simulink model "a6_real_test"  (R2023b)
settings: Solver=FixedStepAuto  StartTime=0.0  StopTime=inf  RelTol=1e-3  EnableMultiTasking=on
undefined symbols (not defined in the file): dev, Main, pwm_output0
libraries: simulink x4, px4Sensorslib x3, px4lib x1, px4uORBlib x1
settings Model: ExtModeTrigDuration=10  Creator=UAV2  LastModifiedBy=UAV2
settings SolverCC: AlgebraicLoopSolver=TrustRegion  PositivePriorityOrder=on  MaxZcPerStep=1
settings OptimizationCC: EnhancedBackFolding=on  PassReuseOutputArgsAs=Individual arguments  ZeroExternalMemoryAtStartup=off  ZeroInternalMemoryAtStartup=off  MaxStackSize=64  OptimizeBlockOrder=speed  DifferentSizesBufferReuse=on  OptimizationCustomize=off  EfficientTunableParamExpr=on
settings DebuggingCC: ParameterTunabilityLossMsg=error  UnconnectedInputMsg=warning  UnconnectedOutputMsg=warning  UnconnectedLineMsg=warning  SymbolicDimsDataTypeCodeGenerationDiagnostic=none
settings HardwareCC: ProdBitPerPointer=32  ProdBitPerSizeT=32  ProdBitPerPtrDiffT=32  ProdLargestAtomicInteger=Long  ProdLargestAtomicFloat=Double  ProdWordSize=32  ProdLongLongMode=on  ProdHWDeviceType=ARM Compatible->ARM Cortex
settings ModelReferenceCC: EnableRefExpFcnMdlSchedulingChecks=on
settings SFSimCC: MATLABDynamicMemAlloc=off  SimTargetLang=C++
settings RTWCC: Description=Embedded Coder  SystemTargetFile=ert.tlc  HardwareBoard=PX4 Pixhawk 4  TLCOptions="-aInlineSetEventsForThisBaseRateFcn=TLC_FALSE -aSuppressMultiTaskScheduler=TLC_FALSE  -aRateBasedStepFcn=0"  TemplateMakefile=ert_default_tmf  Toolchain=GNU Tools for PX4 Autopilots  IncludeHyperlinkInReport=on  TargetLang=C++  DLArmComputeVersion=19.05
settings CodeAppCC: ForceParamTrailComments=on  IgnoreCustomStorageClasses=off  OperatorAnnotations=on  SimulinkDataObjDesc=on  SFDataObjDesc=on  InsertBlockDesc=on
settings ERTTargetCC: ExtModeTransport=3  ExtModeStaticAlloc=on  ExtModeStaticAllocSize=1024  ExtModeMexFile=ext_xcp  ExtModeIntrfLevel=Level2 - Open

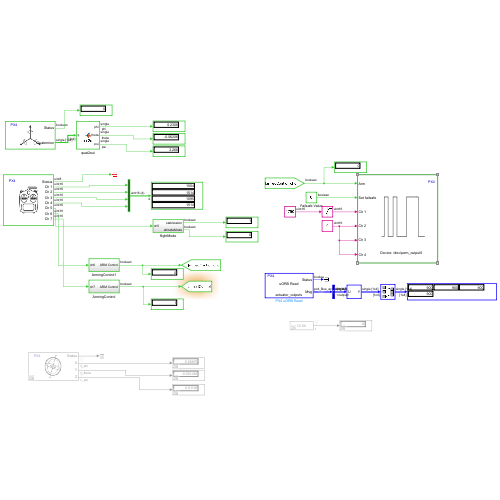
[thumbnail: Simulink's stored preview of the top-level diagram]
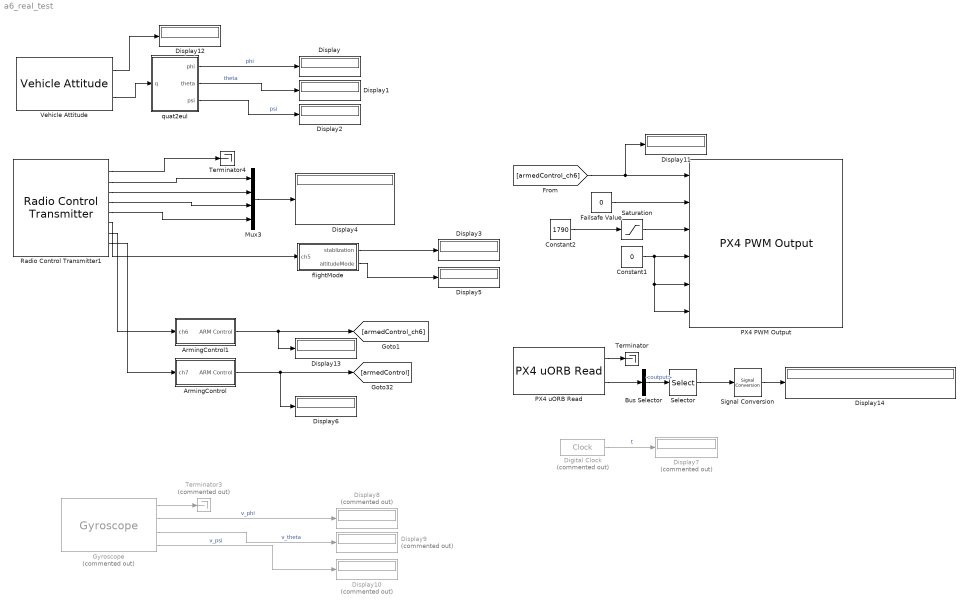
== system a6_real_test ==
  ArmingControl : Subsystem
  ArmingControl1 : Subsystem
  Bus Selector : BusSelector  OutputSignals=output
  Constant1 : Constant  Value=0  OutDataTypeStr=uint16
  Constant2 : Constant  Value=1790  OutDataTypeStr=uint16
  Digital Clock : DigitalClock  Commented=on
  Display{,1..6,11..14} (11 alike) : Display
      Display4 settings: Format=decimal (Stored Integer)
  Display{7..10} (4 alike) : Display  Commented=on
  Failsafe Value : Constant  Value=0  OutDataTypeStr=boolean  SampleTime=-1
  Gyroscope : px4Sensorslib/Gyroscope  Commented=on  uorbTimeStamp=off  BlockingMode=off  BlockTimeout=1e-3  sampleTime=1/250
  Mux3 : Mux
  PX4 PWM Output : px4lib/PX4 PWM Output  pwmDevice=Main (/dev/pwm_output0)  pwmChannel1_=on  pwmChannel2_=on  pwmChannel3_=on  pwmChannel4_=on  pwmChannel5_=off  pwmChannel6_=off  pwmChannel7_=off  pwmChannel8_=off  forceTerminateFailsafe=off  outputErrorStatus=off
  PX4 uORB Read : px4uORBlib/PX4 uORB Read  uORBTopic=actuator_outputs  selectInstance=actuator_outputs  SampleTime=0.01  BlockingMode=off  BlockTimeout=1e-3
  Radio Control Transmitter1 : px4Sensorslib/Radio Control Transmitter  channel1=on  channel2=on  channel3=on  channel4=on  channel5=on  channel6=on  channel7=on  channel8=off  channel_count=off  rssi=off  rc_input_source=off  timestamp_last_signal=off  time_stamp=off  sampleTime=1/250  BlockingMode=off  BlockTimeout=5
  Saturation : Saturate  UpperLimit=2000  LowerLimit=1000
  Selector : Selector  InputPortWidth=16  IndexOptions=Index vector (dialog)  Indices=[1 2 3 4]  OutputSizes=1
  Signal Conversion : SignalConversion  OverrideOpt=off
  Terminator : Terminator
  Terminator3 : Terminator  Commented=on
  Terminator4 : Terminator
  Vehicle Attitude : px4Sensorslib/Vehicle Attitude  rollRate=off  pitchRate=off  yawRate=off  quaternion=on  uorbTimeStamp=off  BlockingMode=off  BlockTimeout=0.001  sampleTime=1/250
  flightMode : Subsystem
  quat2eul : MATLAB Function  TreatAsAtomicUnit=on
  wires:
  Failsafe Value/1 -> PX4 PWM Output/2
  Radio Control Transmitter1/1 -> Terminator4/1
  Mux3/1 -> Display4/1
  Radio Control Transmitter1/2 -> Mux3/1
  Radio Control Transmitter1/3 -> Mux3/2
  Radio Control Transmitter1/4 -> Mux3/3
  Radio Control Transmitter1/5 -> Mux3/4
  Vehicle Attitude/1 -> Display12/1
  quat2eul/2(theta) -> Display1/1  "theta"
  Vehicle Attitude/2 -> quat2eul/1(q)
  quat2eul/1(phi) -> Display/1  "phi"
  quat2eul/3(psi) -> Display2/1  "psi"
  Gyroscope/2 -> Display8/1  "v_phi"
  Gyroscope/1 -> Terminator3/1
  Gyroscope/3 -> Display9/1  "v_theta"
  Gyroscope/4 -> Display10/1  "v_psi"
  Digital Clock/1 -> Display7/1  "t"
  Radio Control Transmitter1/8 -> ArmingControl/1(ch7)
  ArmingControl/1(ARM Control) -> Display6/1, [armedControl]
  Radio Control Transmitter1/6 -> flightMode/1(ch5)
  flightMode/2(altitudeMode) -> Display5/1
  flightMode/1(stablization) -> Display3/1
  Radio Control Transmitter1/7 -> ArmingControl1/1(ch6)
  ArmingControl1/1(ARM Control) -> Display13/1, [armedControl_ch6]
  Signal Conversion/1 -> Display14/1
  PX4 uORB Read/2 -> Bus Selector/1
  Selector/1 -> Signal Conversion/1
  PX4 uORB Read/1 -> Terminator/1
  Bus Selector/1 -> Selector/1  "<output>"
  [armedControl_ch6] -> Display11/1, PX4 PWM Output/1
  Constant2/1 -> Saturation/1
  Constant1/1 -> PX4 PWM Output/5, PX4 PWM Output/6, PX4 PWM Output/4
  Saturation/1 -> PX4 PWM Output/3

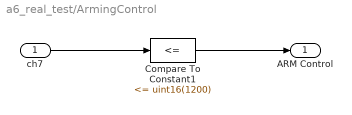
== system a6_real_test/ArmingControl ==
  ch7 : Inport
  Compare To Constant1 : simulink/Logic and Bit Operations/Compare To Constant  relop=<=  const=uint16(1200)  OutDataTypeStr=boolean
  ARM Control : Outport  OutDataTypeStr=boolean  VectorParamsAs1DForOutWhenUnconnected=off
  wires:
  Compare To Constant1/1 -> ARM Control/1
  ch7/1 -> Compare To Constant1/1

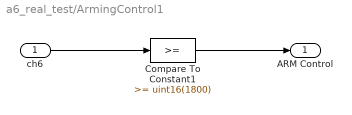
== system a6_real_test/ArmingControl1 ==
  ch6 : Inport
  Compare To Constant1 : simulink/Logic and Bit Operations/Compare To Constant  relop=>=  const=uint16(1800)  OutDataTypeStr=boolean
  ARM Control : Outport  OutDataTypeStr=boolean  VectorParamsAs1DForOutWhenUnconnected=off
  wires:
  ch6/1 -> Compare To Constant1/1
  Compare To Constant1/1 -> ARM Control/1

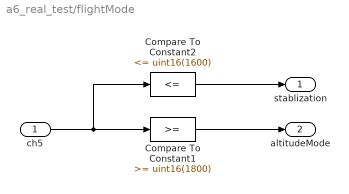
== system a6_real_test/flightMode ==
  ch5 : Inport
  Compare To Constant1 : simulink/Logic and Bit Operations/Compare To Constant  relop=>=  const=uint16(1800)  OutDataTypeStr=boolean
  Compare To Constant2 : simulink/Logic and Bit Operations/Compare To Constant  relop=<=  const=uint16(1600)  OutDataTypeStr=boolean
  stablization : Outport  OutDataTypeStr=boolean  VectorParamsAs1DForOutWhenUnconnected=off
  altitudeMode : Outport  Port=2  OutDataTypeStr=boolean  VectorParamsAs1DForOutWhenUnconnected=off
  wires:
  ch5/1 -> Compare To Constant2/1, Compare To Constant1/1
  Compare To Constant1/1 -> altitudeMode/1
  Compare To Constant2/1 -> stablization/1

== matlab function a6_real_test/quat2eul ==
  data: q input; phi output; theta output; psi output
function [phi,theta,psi] = quat2eul(q)

% Quaternion conversion to Euler angles based on the PX4 Firmware v1.10.2
% release.

phi = atan2(2*(q(1)*q(2) + q(3)* q(4)), q(1)^2 - q(2)^2 - q(3)^2 + q(4)^2);
theta = asin(-2*(q(2)*q(4) - q(1)*q(3)));
psi = atan2(2*(q(2)*q(3) + q(1)* q(4)), q(1)^2 + q(2)^2 - q(3)^2 - q(4)^2);

end
